simulink model "MainProporcional"  (R2021b)
settings: Solver=FixedStepAuto  StartTime=0.0  StopTime=inf  RelTol=1e-3  EnableMultiTasking=on
settings Model: ExtModeTrigDuration=2  Creator=yo  LastModifiedBy=ferna
settings SolverCC: AutoInsertRateTranBlk=on
settings OptimizationCC: EnhancedBackFolding=on  PassReuseOutputArgsAs=Individual arguments  ZeroExternalMemoryAtStartup=off  ZeroInternalMemoryAtStartup=off  MaxStackSize=64  OptimizeBlockOrder=speed  DifferentSizesBufferReuse=on  OptimizationCustomize=off  EfficientTunableParamExpr=on
settings DebuggingCC: MultiTaskRateTransMsg=warning  ParameterTunabilityLossMsg=error
settings HardwareCC: ProdBitPerInt=16  ProdBitPerPointer=16  ProdBitPerSizeT=16  ProdBitPerPtrDiffT=16  ProdLargestAtomicFloat=None  ProdWordSize=8  ProdHWDeviceType=Atmel->AVR  UseEmbeddedCoderFeatures=off  UseSimulinkCoderFeatures=off
settings SFSimCC: MATLABDynamicMemAlloc=off
settings RTWCC: Description=Embedded Coder  SystemTargetFile=ert.tlc  HardwareBoard=Arduino Mega 2560  TemplateMakefile=ert_default_tmf  Toolchain=Arduino AVR  BuildConfiguration=Faster Runs
settings CodeAppCC: ForceParamTrailComments=on  IgnoreCustomStorageClasses=off  OperatorAnnotations=on  SimulinkDataObjDesc=on  SFDataObjDesc=on  MangleLength=10  InsertBlockDesc=on
settings ERTTargetCC: SupportContinuousTime=on  SupportNonInlinedSFcns=on  SupportVariableSizeSignals=on  ExtModeTransport=3  ExtModeStaticAlloc=on  ExtModeStaticAllocSize=2048  ExtModeMexFile=ext_xcp  ExtModeIntrfLevel=Level2 - Open

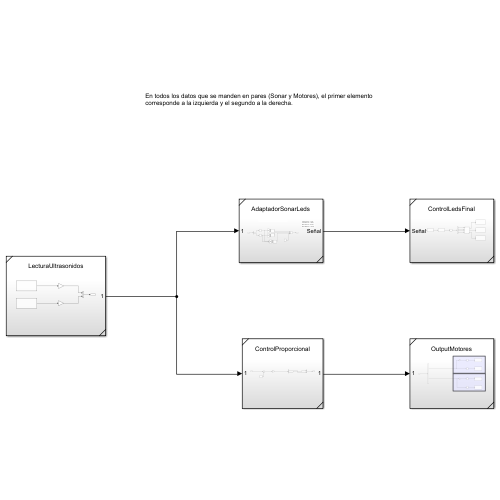
[thumbnail: Simulink's stored preview of the top-level diagram]
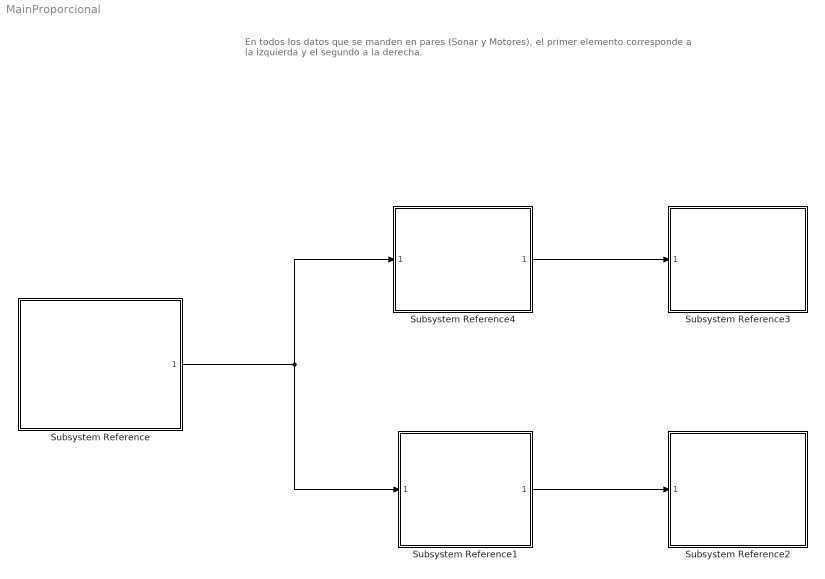
== system MainProporcional ==
  note: En todos los datos que se manden en pares (Sonar y Motores), el primer elemento corresponde a la izquierda y el segundo a la derecha.
  Subsystem Reference : Subsystem  ReferencedSubsystem=LecturaUltrasonidos
  Subsystem Reference1 : Subsystem  ReferencedSubsystem=ControlProporcional
  Subsystem Reference2 : Subsystem  ReferencedSubsystem=OutputMotores
  Subsystem Reference3 : Subsystem  ReferencedSubsystem=ControlLedsFinal
  Subsystem Reference4 : Subsystem  ReferencedSubsystem=AdaptadorSonarLeds
  wires:
  Subsystem Reference/1 -> Subsystem Reference1/1, Subsystem Reference4/1
  Subsystem Reference4/1 -> Subsystem Reference3/1
  Subsystem Reference1/1 -> Subsystem Reference2/1
